simulink model "counter"  (R2021a)
settings: Solver=FixedStepAuto  StartTime=0.0  StopTime=10.0  RelTol=1e-3
model workspace (MAT data in the model file):
  A = 0
  B = 5
settings Model: ParameterArgumentNames=A  OrderedModelArguments=off  Creator=user  LastModifiedBy=user
settings OptimizationCC: DefaultParameterBehavior=Inlined  EnhancedBackFolding=on  PassReuseOutputArgsAs=Individual arguments  ZeroExternalMemoryAtStartup=off  ZeroInternalMemoryAtStartup=off  OptimizeBlockOrder=speed  DifferentSizesBufferReuse=on  OptimizationCustomize=off  EfficientTunableParamExpr=on
settings DebuggingCC: ParameterTunabilityLossMsg=error
settings SFSimCC: MATLABDynamicMemAlloc=off
settings RTWCC: SystemTargetFile=ert.tlc  GenCodeOnly=on  TemplateMakefile=ert_default_tmf  GenerateReport=on  IncludeHyperlinkInReport=on  LaunchReport=on  GenerateTraceInfo=on
settings CodeAppCC: ForceParamTrailComments=on  IgnoreCustomStorageClasses=off  OperatorAnnotations=on  SimulinkDataObjDesc=on  SFDataObjDesc=on  InsertBlockDesc=on
settings ERTTargetCC: TargetLangStandard=C99 (ISO)  GenerateSampleERTMain=on  InlinedParameterPlacement=NonHierarchical  ERTCustomFileTemplate=example_file_process.tlc

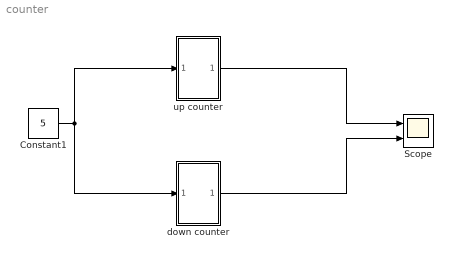
== system counter ==
  Constant1 : Constant  Value=5
  Scope : Scope  NumInputPorts=2
  down counter : Subsystem
  up counter : Subsystem
  wires:
  Constant1/1 -> down counter/1(In1), up counter/1(In1)
  up counter/1(Out1) -> Scope/1
  down counter/1(Out1) -> Scope/2

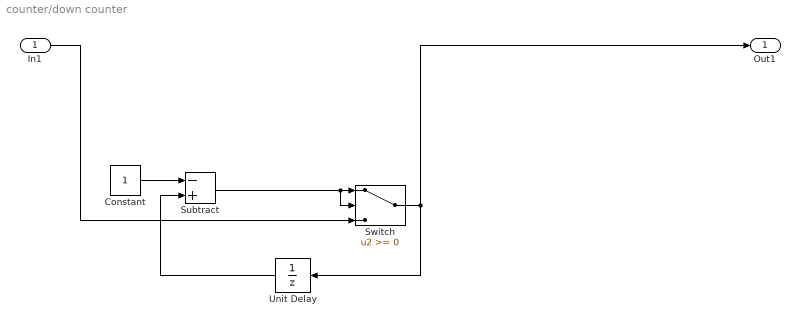
== system counter/down counter ==
  In1 : Inport
  Constant : Constant
  Subtract : Sum  Inputs=-+
  Switch : Switch
  Unit Delay : UnitDelay  SampleTime=-1  HasFrameUpgradeWarning=on
  Out1 : Outport
  wires:
  In1/1 -> Switch/3
  Subtract/1 -> Switch/2, Switch/1
  Constant/1 -> Subtract/1
  Switch/1 -> Out1/1, Unit Delay/1
  Unit Delay/1 -> Subtract/2

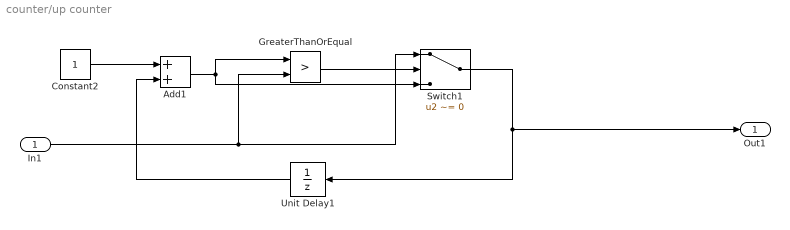
== system counter/up counter ==
  In1 : Inport
  Add1 : Sum
  Constant2 : Constant
  GreaterThanOrEqual : RelationalOperator  Operator=>  OutDataTypeStr=boolean  RndMeth=Simplest
  Switch1 : Switch  Criteria=u2 ~= 0
  Unit Delay1 : UnitDelay  InitialCondition=-1  HasFrameUpgradeWarning=on
  Out1 : Outport
  wires:
  In1/1 -> Switch1/1, GreaterThanOrEqual/2
  Add1/1 -> Switch1/3, GreaterThanOrEqual/1
  Constant2/1 -> Add1/1
  GreaterThanOrEqual/1 -> Switch1/2
  Switch1/1 -> Out1/1, Unit Delay1/1
  Unit Delay1/1 -> Add1/2
